simulink model "problem2_1"  (R2016a)
settings: Solver=VariableStepAuto  StartTime=0.0  StopTime=10  RelTol=1e-3  SampleTimeConstraint=Specified
values from neighbouring files (symbols this model uses):
  D = B*0    [main.m]
  x2_i = [0.3;0.45]    [main.m]    (also in main_1.m = IK()
  x_path = planTraj(x2_i(1),x2_f(1),time)    [main.m]    (also in main_1.m = planTraj(x2_i(1),x2_f(1), 3))
  y_path = planTraj(x2_i(2),x2_f(2),time)    [main.m]    (also in main_1.m = planTraj(x2_i(2),x2_f(2),3))
libraries: dspinverses x1
settings Model: Creator=nathaniel  LastModifiedBy=nathaniel
settings GRTTargetCC: GeneratePreprocessorConditionals=Use local settings

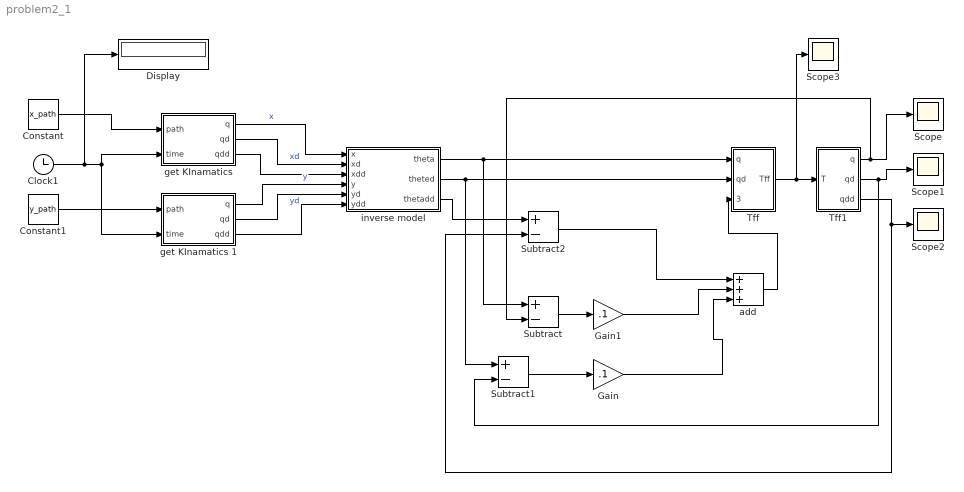
== system problem2_1 ==
  Clock1 : Clock
  Constant : Constant  Value=x_path
  Constant1 : Constant  Value=y_path
  Display : Display
  Gain : Gain  Gain=.1
  Gain1 : Gain  Gain=.1
  Scope{,1..3} (4 alike) : Scope
  Subtract : Sum  Inputs=+-
  Subtract1 : Sum  Inputs=+-
  Subtract2 : Sum  Inputs=+-
  Tff : Subsystem
  Tff1 : Subsystem
  "add " : Sum  Inputs=+++
  "get KInamatics " : MATLAB Function  TreatAsAtomicUnit=on
  get KInamatics 1 : MATLAB Function  TreatAsAtomicUnit=on
  inverse model : Subsystem
  wires:
  Clock1/1 -> Display/1, "get KInamatics "/2(time), get KInamatics 1/2(time)
  Constant1/1 -> get KInamatics 1/1(path)
  Constant/1 -> "get KInamatics "/1(path)
  "get KInamatics "/1(q) -> inverse model/1(x)  "x"
  "get KInamatics "/2(qd) -> inverse model/2(xd)  "xd"
  "get KInamatics "/3(qdd) -> inverse model/3(xdd)
  get KInamatics 1/1(q) -> inverse model/4(y)  "y"
  get KInamatics 1/2(qd) -> inverse model/5(yd)  "yd"
  get KInamatics 1/3(qdd) -> inverse model/6(ydd)
  inverse model/1(theta) -> Subtract/1, Tff/1(q)
  inverse model/2(theted) -> Subtract1/1, Tff/2(qd)
  Tff1/1(q) -> Subtract/2, Scope/1
  Tff1/3(qdd) -> Subtract2/2, Scope2/1
  Tff/1(Tff) -> Scope3/1, Tff1/1(T)
  Tff1/2(qd) -> Subtract1/2, Scope1/1
  Subtract/1 -> Gain1/1
  "add "/1 -> Tff/3(qdd)
  inverse model/3(thetadd) -> Subtract2/1
  Subtract1/1 -> Gain/1
  Gain1/1 -> "add "/2
  Subtract2/1 -> "add "/1
  Gain/1 -> "add "/3

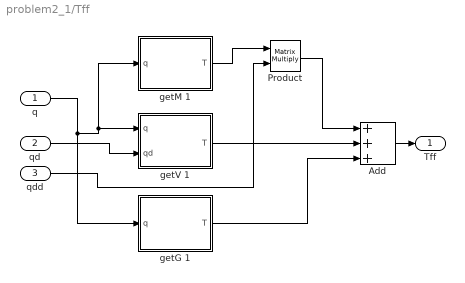
== system problem2_1/Tff ==
  q : Inport
  qd : Inport  Port=2
  qdd : Inport  Port=3
  Add : Sum  Inputs=+++
  Product : Product  Multiplication=Matrix(*)
  getG 1 : MATLAB Function  TreatAsAtomicUnit=on
  getM 1 : MATLAB Function  TreatAsAtomicUnit=on
  getV 1 : MATLAB Function  TreatAsAtomicUnit=on
  Tff : Outport
  wires:
  q/1 -> getG 1/1(q), getV 1/1(q), getM 1/1(q)
  qdd/1 -> Product/2
  Add/1 -> Tff/1
  Product/1 -> Add/1
  getM 1/1(T) -> Product/1
  getG 1/1(T) -> Add/3
  qd/1 -> getV 1/2(qd)
  getV 1/1(T) -> Add/2

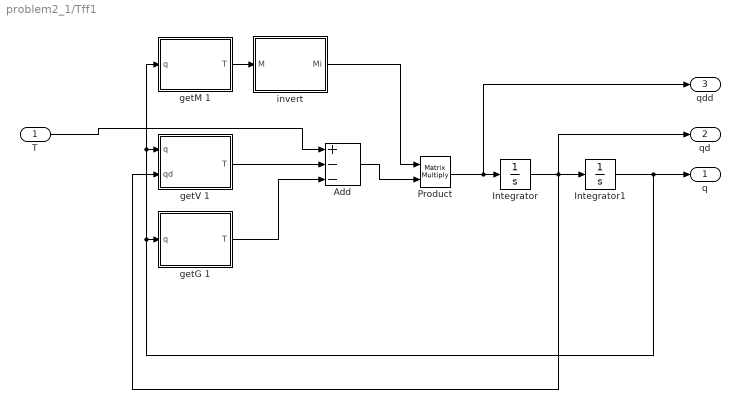
== system problem2_1/Tff1 ==
  T : Inport
  Add : Sum  Inputs=+--
  Integrator : Integrator  InitialCondition=[0;0]
  Integrator1 : Integrator  InitialCondition=x2_i
  Product : Product  Multiplication=Matrix(*)
  getG 1 : MATLAB Function  TreatAsAtomicUnit=on
  getM 1 : MATLAB Function  TreatAsAtomicUnit=on
  getV 1 : MATLAB Function  TreatAsAtomicUnit=on
  invert : MATLAB Function  TreatAsAtomicUnit=on
  q : Outport
  qd : Outport  Port=2
  qdd : Outport  Port=3
  wires:
  getV 1/1(T) -> Add/2
  getG 1/1(T) -> Add/3
  T/1 -> Add/1
  getM 1/1(T) -> invert/1(M)
  invert/1(Mi) -> Product/1
  Add/1 -> Product/2
  Integrator/1 -> getV 1/2(qd), qd/1, Integrator1/1
  Integrator1/1 -> getM 1/1(q), getV 1/1(q), getG 1/1(q), q/1
  Product/1 -> qdd/1, Integrator/1

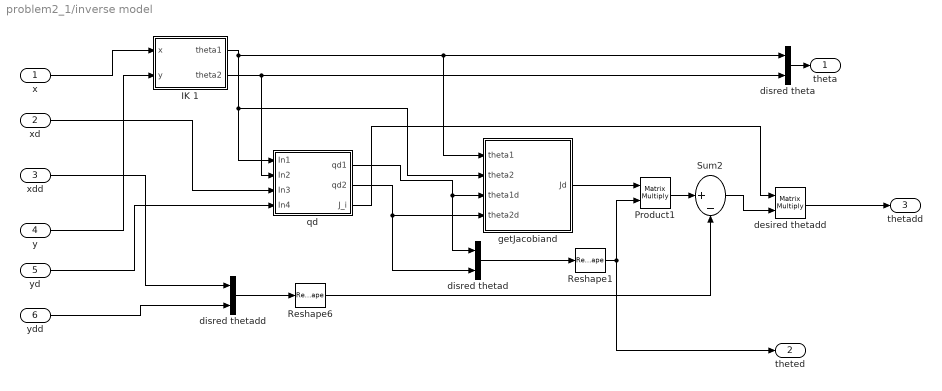
== system problem2_1/inverse model ==
  x : Inport
  xd : Inport  Port=2
  xdd : Inport  Port=3
  y : Inport  Port=4
  yd : Inport  Port=5
  ydd : Inport  Port=6
  IK 1 : MATLAB Function  TreatAsAtomicUnit=on
  Product1 : Product  Multiplication=Matrix(*)
  Reshape1 : Reshape  OutputDimensionality=Column vector (2-D)
  Reshape6 : Reshape  OutputDimensionality=Column vector (2-D)
  Sum2 : Sum  Inputs=|+-
  desired thetadd : Product  Multiplication=Matrix(*)
  disred theta : Concatenate
  disred thetad : Concatenate
  "disred thetadd " : Concatenate
  "getJacobiand " : MATLAB Function  TreatAsAtomicUnit=on
  qd : Subsystem
  theta : Outport
  theted : Outport  Port=2
  thetadd : Outport  Port=3
  wires:
  Reshape6/1 -> Sum2/2
  qd/1(qd1) -> disred thetad/1, "getJacobiand "/3(theta1d)
  "getJacobiand "/1(Jd) -> Product1/1
  qd/2(qd2) -> "getJacobiand "/4(theta2d), disred thetad/2
  disred thetad/1 -> Reshape1/1
  Sum2/1 -> desired thetadd/2
  Product1/1 -> Sum2/1
  disred theta/1 -> theta/1
  xd/1 -> qd/3(In3)
  IK 1/2(theta2) -> disred theta/2, qd/2(In2)
  "disred thetadd "/1 -> Reshape6/1
  yd/1 -> qd/4(In4)
  desired thetadd/1 -> thetadd/1
  Reshape1/1 -> Product1/2, theted/1
  x/1 -> IK 1/1(x)
  ydd/1 -> "disred thetadd "/2
  xdd/1 -> "disred thetadd "/1
  y/1 -> IK 1/2(y)
  qd/3(J_i) -> desired thetadd/1
  IK 1/1(theta1) -> "getJacobiand "/1(theta1), disred theta/1, "getJacobiand "/2(theta2), qd/1(In1)

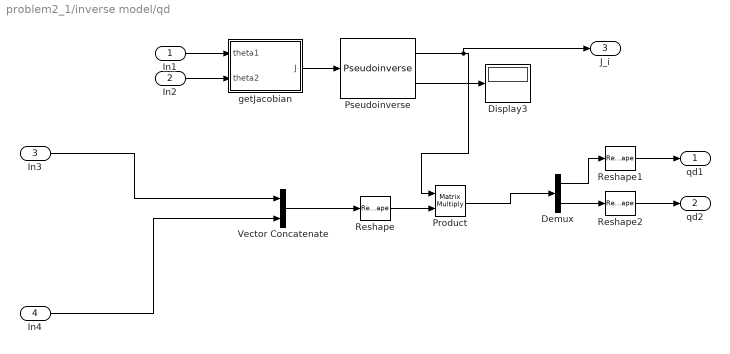
== system problem2_1/inverse model/qd ==
  In1 : Inport
  In2 : Inport  Port=2
  In3 : Inport  Port=3
  In4 : Inport  Port=4
  Demux : Demux  Outputs=2
  Display3 : Display
  Product : Product  Multiplication=Matrix(*)
  Pseudoinverse : dspinverses/Pseudoinverse  wanterr=on
  Reshape : Reshape  OutputDimensionality=Column vector (2-D)
  Reshape1 : Reshape  OutputDimensionality=Customize  OutputDimensions=1
  Reshape2 : Reshape  OutputDimensionality=Customize  OutputDimensions=1
  Vector Concatenate : Concatenate
  getJacobian : MATLAB Function  TreatAsAtomicUnit=on
  qd1 : Outport
  qd2 : Outport  Port=2
  J_i : Outport  Port=3
  wires:
  Pseudoinverse/2 -> Display3/1
  getJacobian/1(J) -> Pseudoinverse/1
  In4/1 -> Vector Concatenate/2
  In3/1 -> Vector Concatenate/1
  Pseudoinverse/1 -> J_i/1, Product/1
  Vector Concatenate/1 -> Reshape/1
  In2/1 -> getJacobian/2(theta2)
  Reshape/1 -> Product/2
  In1/1 -> getJacobian/1(theta1)
  Product/1 -> Demux/1
  Demux/2 -> Reshape2/1
  Demux/1 -> Reshape1/1
  Reshape1/1 -> qd1/1
  Reshape2/1 -> qd2/1

== matlab function problem2_1/get KInamatics 1 ==
  data: path input; q output; time input; qd output; qdd output
function [ q,qd,qdd] = fcn(path, time)
%#codegen
[q qd qdd] = getKin(path, time);

== matlab function problem2_1/get KInamatics  ==
  data: path input; q output; time input; qd output; qdd output
function [ q,qd,qdd] = fcn(path, time)
%#codegen
[q qd qdd] = getKin(path, time);

== matlab function problem2_1/inverse model/getJacobiand  ==
  data: theta1 input; theta2 input; theta1d input; Jd output; theta2d input
function Jd  = fcn(theta1,theta2, theta1d, theta2d)
%#codegen
Jd = getJacobiandot(theta1,theta1d,theta2,theta2d);

== matlab function problem2_1/inverse model/IK 1 ==
  data: x input; theta1 output; y input; theta2 output
function [ theta1, theta2] = fcn(x, y)
%#codegen
[theta1 theta2] = IK(x, y);

== matlab function problem2_1/inverse model/qd/getJacobian ==
  data: theta1 input; J output; theta2 input
function J  = fcn(theta1, theta2)
%#codegen
J = getJacobian(theta1,theta2);

== matlab function problem2_1/Tff/getM 1 ==
  data: q input; T output
function T = fcn(q)
%#codegen
T = getM(q);

== matlab function problem2_1/Tff/getV 1 ==
  data: q input; T output; qd input
function T = fcn(q, qd)
%#codegen
T = getV(q, qd);

== matlab function problem2_1/Tff/getG 1 ==
  data: q input; T output
function T = fcn(q)
%#codegen
T = getG(q);

== matlab function problem2_1/Tff1/getG 1 ==
  data: q input; T output
function T = fcn(q)
%#codegen
T = getG(q);

== matlab function problem2_1/Tff1/getM 1 ==
  data: q input; T output
function T = fcn(q)
%#codegen
T = getM(q);

== matlab function problem2_1/Tff1/getV 1 ==
  data: q input; T output; qd input
function T = fcn(q, qd)
%#codegen
T = getV(q, qd);

== matlab function problem2_1/Tff1/invert ==
  data: M input; Mi output
function Mi = fcn(M)
%#codegen
Mi =pinv(M);
